simulink model "semi_withrl"  (R2013b)
settings: Solver=ode45  StartTime=0.0  StopTime=0.08  RelTol=1e-3
undefined symbols (not defined in the file): alpha
libraries: powerlib x12, powerlib_meascontrol x2
settings Model: Creator=SAI KUMAR  LastModifiedBy=SAI KUMAR

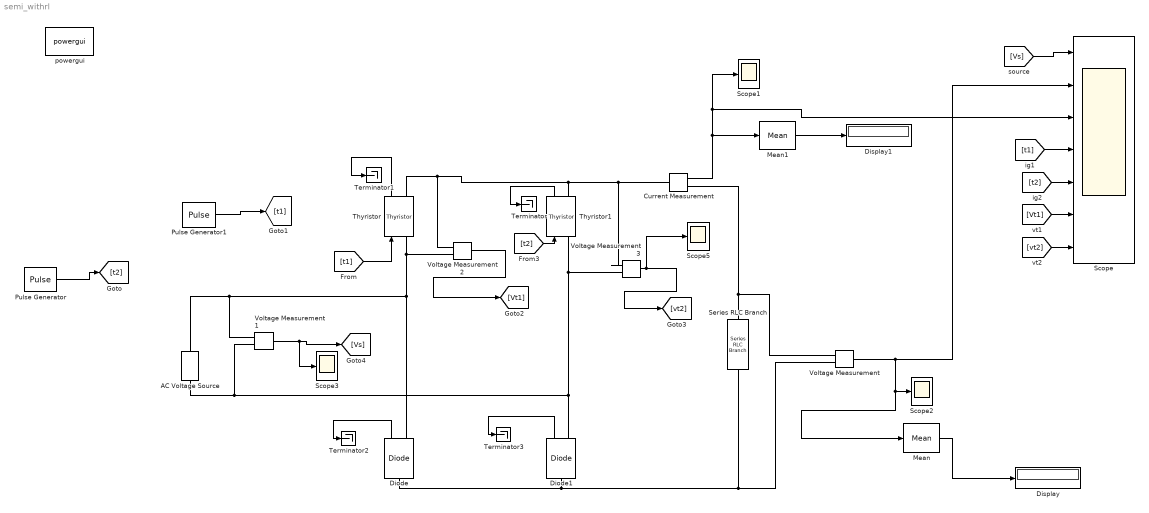
== system semi_withrl ==
  AC Voltage Source : powerlib/Electrical Sources/AC Voltage Source  Amplitude=220*sqrt(2)  Phase=0  Frequency=50  SampleTime=0  Measurements=None
  Current Measurement : powerlib/Measurements/Current Measurement  PhasorSimulation=off  OutputType=Complex  PSBequivalent=0
  Diode : powerlib/Power Electronics/Diode  Ron=0.001  Lon=0  Vf=0.8  IC=0  UseSnubber=off  Rs=500  Cs=250e-9  Measurements=on
  Diode1 : powerlib/Power Electronics/Diode  Ron=0.001  Lon=0  Vf=0.8  IC=0  UseSnubber=off  Rs=500  Cs=250e-9  Measurements=on
  Display : Display
  Display1 : Display
  Mean : powerlib_meascontrol/Measurements/Mean  Freq=60  Vinit=0  Ts=0
  Mean1 : powerlib_meascontrol/Measurements/Mean  Freq=60  Vinit=0  Ts=0
  Pulse Generator : DiscretePulseGenerator  PulseType=Time based  Amplitude=5  Period=0.02  PulseWidth=10  PhaseDelay=(0.02/360)*alpha+0.01
  Pulse Generator1 : DiscretePulseGenerator  PulseType=Time based  Amplitude=5  Period=0.02  PulseWidth=10  PhaseDelay=(0.02/360)*alpha
  Scope : Scope  NumInputPorts=7
      settings: TickLabels=on  ShowLegends=on  TimeRange=0.08  YMin=-400~-2~-0.2~0~0~-400~-400  YMax=400~6~0.6000000000000001~6~6~200~200  SampleInput=on
  Scope{1..3,5} (4 alike) : Scope
      Scope1 settings: TimeRange=5  YMin=5  YMax=85  SampleInput=on
      Scope2 settings: TimeRange=5  YMin=5  YMax=85  SaveName=ScopeData2  SampleInput=on
      Scope3 settings: TimeRange=5  YMin=5  YMax=85  SaveName=ScopeData3  SampleInput=on
      Scope5 settings: TimeRange=5  YMin=5  YMax=85  SaveName=ScopeData4  SampleInput=on
  Series RLC Branch : powerlib/Elements/Series RLC Branch  LConnTagsString=__new0  RConnTagsString=__new0  BranchType=RL  Resistance=60  Inductance=0.5  SetiL0=off  InitialCurrent=0  Capacitance=1e-6  Setx0=off  InitialVoltage=0  Measurements=None
  Terminator{,1..3} (4 alike) : Terminator
  Thyristor : powerlib/Power Electronics/Thyristor  Ron=0.001  Lon=0  Vf=0.8  IC=0  Rs=500  Cs=250e-9  Measurements=on
  Thyristor1 : powerlib/Power Electronics/Thyristor  Ron=0.001  Lon=0  Vf=0.8  IC=0  Rs=500  Cs=250e-9  Measurements=on
  Voltage Measurement{,1..3} (4 alike) : powerlib/Measurements/Voltage Measurement  PhasorSimulation=off  OutputType=Complex  PSBequivalent=0
  powergui : powerlib/powergui  Priority=1  SimulationMode=Continuous  SolverType=Tustin  SampleTime=50e-6  frequency=60  SPID=off  DisableSnubberDevices=off  DisableRonSwitches=off  DisableVfSwitches=off  SwTol=0  Interpol=off  DisplayEquations=off  frequencyindice=50  Pbase=100e6  ErrMax=1e-4  Iterations=50  UnitsV=kV  UnitsW=MW  FunctionMessages=off  echomessages=off  HookPort=off  EnableUseOfTLC=off  x0status=blocks  RestoreLinks=warning  ResistiveCurrentMeasurement=off  Frange=[0:2:500]  Ylog=off  Xlog=on  ShowGrid=off  save=off  variable=ZData  ZoomFFT=off  StartTime=0.0  cycles=1  DisplayStyle=1  fundamental=60  FreqAxis=off  MaxFrequency=1000  frequencyindicesteady=1  RmsSteady=1  display=off  Ts=0  methode=off
  wires:
  Pulse Generator/1 -> [t2]
  Pulse Generator1/1 -> [t1]
  Current Measurement/1 -> Scope1/1, Scope/3, Mean1/1
  Voltage Measurement/1 -> Mean/1, Scope2/1, Scope/2
  [t2] -> Thyristor1/1
  Mean/1 -> Display/1
  Voltage Measurement1/1 -> Scope3/1, [Vs]
  Thyristor1/1 -> Terminator/1
  Thyristor/1 -> Terminator1/1
  Voltage Measurement3/1 -> Scope5/1, [vt2]
  [vt2] -> Scope/7
  [t1] -> Thyristor/1
  Voltage Measurement2/1 -> [Vt1]
  Mean1/1 -> Display1/1
  [Vs] -> Scope/1
  [Vt1] -> Scope/6
  [t2] -> Scope/5
  [t1] -> Scope/4
  Diode1/1 -> Terminator3/1
  Diode/1 -> Terminator2/1
  connections:
  Voltage Measurement/LConn1 -- Current Measurement/RConn1 -- Series RLC Branch/LConn1
  Diode/RConn1 -- Thyristor/LConn1 -- Voltage Measurement2/LConn2 -- Voltage Measurement1/LConn1 -- AC Voltage Source/RConn1
  Current Measurement/LConn1 -- Voltage Measurement3/LConn1 -- Thyristor1/RConn1 -- Thyristor/RConn1 -- Voltage Measurement2/LConn1
  Thyristor1/LConn1 -- Voltage Measurement3/LConn2 -- Diode1/RConn1 -- Voltage Measurement1/LConn2 -- AC Voltage Source/LConn1
  Diode1/LConn1 -- Series RLC Branch/RConn1 -- Voltage Measurement/LConn2 -- Diode/LConn1
